simulink model "MoPhongXe2BanhCanBang_LQR"  (R2022b)
settings: Solver=VariableStepAuto  StartTime=0.0  StopTime=100  RelTol=1e-3
values from neighbouring files (symbols this model uses):
  K = lqr(A,B,Q,R__)    [CacFunctionTrongSimulink_LQR.m]
  x1_init = 0.001    [CacFunctionTrongSimulink_LQR.m]
  x2_init = -0.0012    [CacFunctionTrongSimulink_LQR.m]
  x4_init = 0.002    [CacFunctionTrongSimulink_LQR.m]
  x5_init = -0.002    [CacFunctionTrongSimulink_LQR.m]
  x7_init = 0.002    [CacFunctionTrongSimulink_LQR.m]
  x8_init = -0.0014    [CacFunctionTrongSimulink_LQR.m]
settings Model: Creator=Administrator  LastModifiedBy=vanph
settings SolverCC: AlgebraicLoopSolver=TrustRegion
settings DebuggingCC: UnconnectedInputMsg=warning  UnconnectedOutputMsg=warning  UnconnectedLineMsg=warning  SFMachineParentedDataDiag=warning  ArithmeticOperatorsInVariantConditions=warning
settings ModelReferenceCC: EnableRefExpFcnMdlSchedulingChecks=on
settings SFSimCC: CustomCodeUndefinedFunction=UseInterfaceOnly

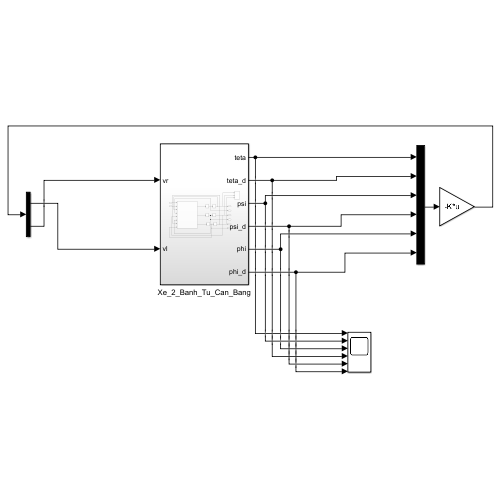
[thumbnail: Simulink's stored preview of the top-level diagram]
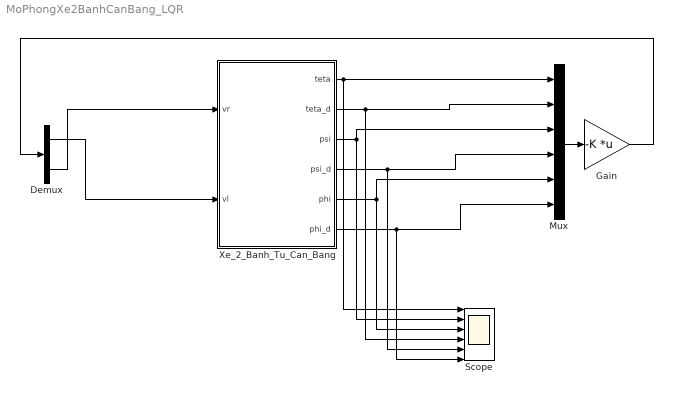
== system MoPhongXe2BanhCanBang_LQR ==
  Demux : Demux  Outputs=2
  Gain : Gain  Gain=-K  Multiplication=Matrix(K*u)
  Mux : Mux  Inputs=6
  Scope : Scope  NumInputPorts=6
  Xe_2_Banh_Tu_Can_Bang : Subsystem
  wires:
  Mux/1 -> Gain/1
  Xe_2_Banh_Tu_Can_Bang/2(teta_d) -> Scope/4, Mux/2
  Xe_2_Banh_Tu_Can_Bang/4(psi_d) -> Scope/5, Mux/4
  Xe_2_Banh_Tu_Can_Bang/6(phi_d) -> Scope/6, Mux/6
  Gain/1 -> Demux/1
  Xe_2_Banh_Tu_Can_Bang/1(teta) -> Mux/1, Scope/1
  Xe_2_Banh_Tu_Can_Bang/3(psi) -> Scope/2, Mux/3
  Xe_2_Banh_Tu_Can_Bang/5(phi) -> Mux/5, Scope/3
  Demux/2 -> Xe_2_Banh_Tu_Can_Bang/1(vr)
  Demux/1 -> Xe_2_Banh_Tu_Can_Bang/2(vl)

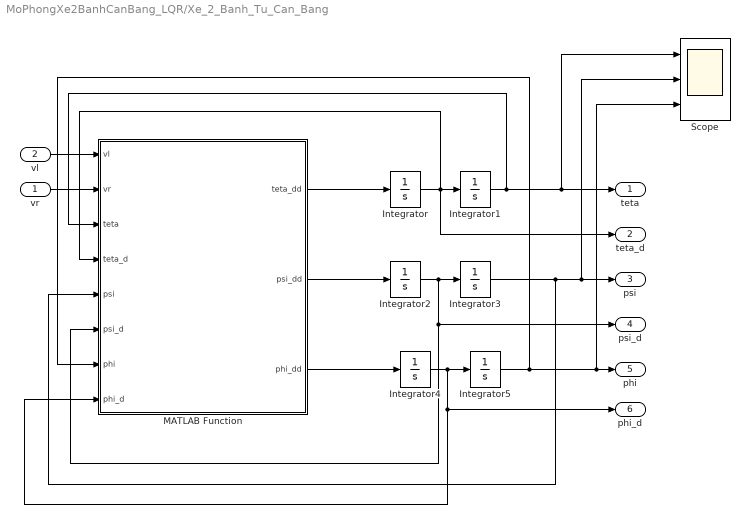
== system MoPhongXe2BanhCanBang_LQR/Xe_2_Banh_Tu_Can_Bang ==
  vr : Inport
  vl : Inport  Port=2
  Integrator : Integrator  InitialCondition=x2_init
  Integrator1 : Integrator  InitialCondition=x1_init
  Integrator2 : Integrator  InitialCondition=x5_init
  Integrator3 : Integrator  InitialCondition=x4_init
  Integrator4 : Integrator  InitialCondition=x8_init
  Integrator5 : Integrator  InitialCondition=x7_init
  MATLAB Function : MATLAB Function  TreatAsAtomicUnit=on
  Scope : Scope  NumInputPorts=3
  teta : Outport
  teta_d : Outport  Port=2
  psi : Outport  Port=3
  psi_d : Outport  Port=4
  phi : Outport  Port=5
  phi_d : Outport  Port=6
  wires:
  Integrator/1 -> MATLAB Function/4(teta_d), Integrator1/1, teta_d/1
  Integrator1/1 -> MATLAB Function/3(teta), Scope/1, teta/1
  MATLAB Function/1(teta_dd) -> Integrator/1
  Integrator3/1 -> MATLAB Function/5(psi), Scope/2, psi/1
  Integrator2/1 -> MATLAB Function/6(psi_d), psi_d/1, Integrator3/1
  MATLAB Function/2(psi_dd) -> Integrator2/1
  Integrator5/1 -> MATLAB Function/7(phi), Scope/3, phi/1
  Integrator4/1 -> MATLAB Function/8(phi_d), phi_d/1, Integrator5/1
  MATLAB Function/3(phi_dd) -> Integrator4/1
  vr/1 -> MATLAB Function/2(vr)
  vl/1 -> MATLAB Function/1(vl)

== matlab function MoPhongXe2BanhCanBang_LQR/Xe_2_Banh_Tu_Can_Bang/MATLAB Function ==
  data: vl input; teta_dd output; vr input; teta input; teta_d input; psi input; psi_d input; phi input; phi_d input; psi_dd output; phi_dd output
function [teta_dd,psi_dd,phi_dd] = fcn(vl,vr,teta,teta_d,psi,psi_d,phi,phi_d)

%% Thông số hệ thống xe 2 bánh tự cân bằng dùng LQR
m = 0.0345; %Khoi luong banh xe
M = 0.875; %Khoi luong robot
R = 0.0325; %ban kinh ban xe
W = 0.225; %Chieu rong robot
D = 0.084; %Chieu sau robot
H = 0.132; %Chieu cao robot
L = 0.091; %khoang cach tu trong tam den truc banh xe
fw = 0.18; %He so ma sat giua banh xe voi mat phang
fm = 0.002; %he so ma sat giua dong co va robot
Jm = 0.000082; %moment quan tinh cua dong co
Jw = m*R^2/2;
J_psi = M*L^2/3;
J_phi = M*(W^2+D^2)/12;
Rm = 13; %Dien tro dong co DC
Kb = 1.91; %he so emf cua dong co
Kt = 0.216 ; %Momen xoan cua dong co DC
n = 33.64; %Ty so giam toc
g = 9.81; %Gia toc trong truong
alpha = n*Kt/Rm; beta=n*Kt*Kb/Rm+fm; a =alpha;
T=0.01;

teta_dd = (J_psi*a*vl + J_psi*a*vr - 2*J_psi*beta*teta_d + 2*J_psi*beta*psi_d - 2*J_psi*fw*teta_d + L^2*M*a*vl + L^2*M*a*vr - 2*L^2*M*beta*teta_d + 2*L^2*M*beta*psi_d - 2*L^2*M*fw*teta_d - 4*Jm*fw*n^2*teta_d + L^3*M^2*R*psi_d^2*sin(psi) - 2*L*M*R*beta*teta_d*cos(psi) + 2*L*M*R*beta*psi_d*cos(psi) - L^3*M^2*R*phi_d^2*cos(psi)^2*sin(psi) - L^2*M^2*R*g*cos(psi)*sin(psi) + J_psi*L*M*R*psi_d^2*sin(psi) + 2*Jm*L*M*g*n^2*sin(psi) + L*M*R*a*vl*cos(psi) + L*M*R*a*vr*cos(psi) + 2*Jm*L^2*M*n^2*phi_d^2*cos(psi)*sin(psi) + 2*Jm*L*M*R*n^2*psi_d^2*sin(psi))/(2*J_psi*Jw + L^2*M^2*R^2 + 2*Jw*L^2*M + J_psi*M*R^2 + 2*J_psi*Jm*n^2 + 4*Jm*Jw*n^2 + 2*J_psi*R^2*m + 2*Jm*L^2*M*n^2 + 2*Jm*M*R^2*n^2 + 2*L^2*M*R^2*m + 4*Jm*R^2*m*n^2 - L^2*M^2*R^2*cos(psi)^2 + 4*Jm*L*M*R*n^2*cos(psi));
psi_dd = -(2*Jw*a*vl + 2*Jw*a*vr - 4*Jw*beta*teta_d + 4*Jw*beta*psi_d + M*R^2*a*vl + M*R^2*a*vr - 2*M*R^2*beta*teta_d + 2*M*R^2*beta*psi_d + 2*R^2*a*m*vl + 2*R^2*a*m*vr + 4*Jm*fw*n^2*teta_d - 4*R^2*beta*m*teta_d + 4*R^2*beta*m*psi_d - L*M^2*R^2*g*sin(psi) - 2*Jw*L*M*g*sin(psi) - 2*L*M*R*beta*teta_d*cos(psi) + 2*L*M*R*beta*psi_d*cos(psi) - 2*L*M*R*fw*teta_d*cos(psi) + L^2*M^2*R^2*psi_d^2*cos(psi)*sin(psi) - L^2*M^2*R^2*phi_d^2*cos(psi)*sin(psi) - 2*Jw*L^2*M*phi_d^2*cos(psi)*sin(psi) - 2*Jm*L*M*g*n^2*sin(psi) - 2*L*M*R^2*g*m*sin(psi) + L*M*R*a*vl*cos(psi) + L*M*R*a*vr*cos(psi) - 2*Jm*L^2*M*n^2*phi_d^2*cos(psi)*sin(psi) - 2*L^2*M*R^2*m*phi_d^2*cos(psi)*sin(psi) - 2*Jm*L*M*R*n^2*psi_d^2*sin(psi))/(2*J_psi*Jw + L^2*M^2*R^2 + 2*Jw*L^2*M + J_psi*M*R^2 + 2*J_psi*Jm*n^2 + 4*Jm*Jw*n^2 + 2*J_psi*R^2*m + 2*Jm*L^2*M*n^2 + 2*Jm*M*R^2*n^2 + 2*L^2*M*R^2*m + 4*Jm*R^2*m*n^2 - L^2*M^2*R^2*cos(psi)^2 + 4*Jm*L*M*R*n^2*cos(psi));
phi_dd = -(W^2*beta*phi_d + W^2*fw*phi_d + R*W*a*vl - R*W*a*vr + 4*L^2*M*R^2*psi_d*phi_d*cos(psi)*sin(psi))/(2*J_phi*R^2 + Jm*W^2 + Jm*W^2*n^2 + R^2*W^2*m + 2*L^2*M*R^2*sin(psi)^2);
